simulink model "t2_2_Dinamica_proyectil"  (R2024a)
settings: Solver=VariableStepAuto  StartTime=0.0  StopTime=7  RelTol=1e-3
settings Model: Creator=scpmoxxa  LastModifiedBy=pablo
settings OptimizationCC: ReuseModelBlockBuffer=off
settings DebuggingCC: UnconnectedInputMsg=warning  UnconnectedOutputMsg=warning  UnconnectedLineMsg=warning
settings ModelReferenceCC: EnableRefExpFcnMdlSchedulingChecks=on
settings RTWCC: GPUComputeCapability=3.5  DLArmComputeVersion=19.05

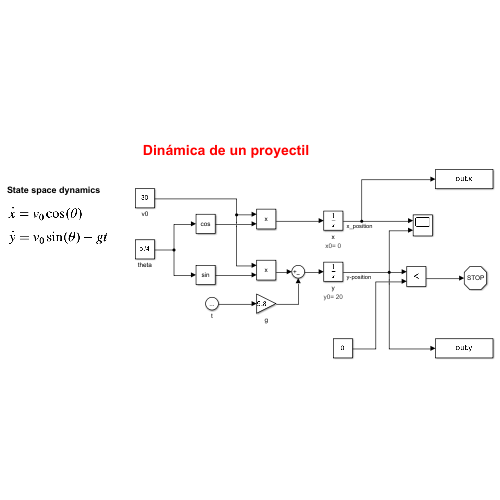
[thumbnail: Simulink's stored preview of the top-level diagram]
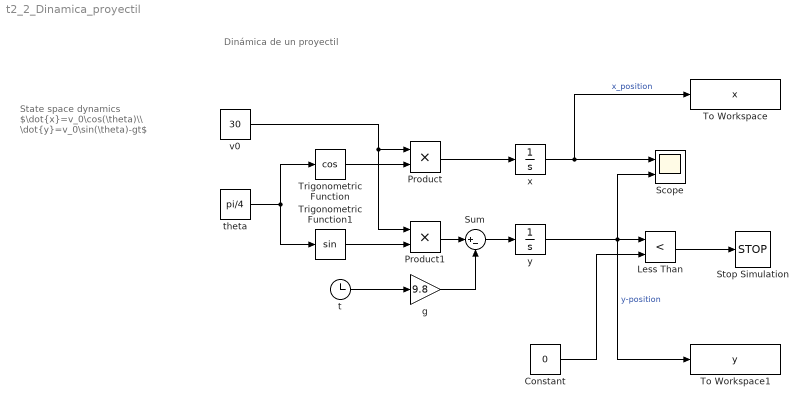
== system t2_2_Dinamica_proyectil ==
  note: State space dynamics
      |
      | $\dot{x}=v_0\cos(\theta)\\ \dot{y}=v_0\sin(\theta)-gt$
  note: Dinámica de un proyectil
  Constant : Constant  Value=0
  Less Than : RelationalOperator  Operator=<  OutDataTypeStr=boolean  RndMeth=Simplest  InputSameDT=off
  Product : Product
  Product1 : Product
  Scope : Scope  NumInputPorts=2
  Stop Simulation : Stop
  Sum : Sum  Inputs=|+-
  To Workspace : ToWorkspace  VariableName=x  SampleTime=-1
  To Workspace1 : ToWorkspace  VariableName=y  SampleTime=-1
  Trigonometric Function : Trigonometry  Operator=cos
  Trigonometric Function1 : Trigonometry
  g : Gain  Gain=9.8
  t : Clock
  theta : Constant  Value=pi/4
  v0 : Constant  Value=30
  x : Integrator
      settings: AttributesFormatString=x0= %<InitialCondition>
  y : Integrator  InitialCondition=20
      settings: AttributesFormatString=y0= %<InitialCondition>
  wires:
  theta/1 -> Trigonometric Function/1, Trigonometric Function1/1
  Trigonometric Function/1 -> Product/2
  v0/1 -> Product1/1, Product/1
  Trigonometric Function1/1 -> Product1/2
  Product/1 -> x/1
  Product1/1 -> Sum/1
  Sum/1 -> y/1
  t/1 -> g/1
  g/1 -> Sum/2
  y/1 -> To Workspace1/1, Scope/2, Less Than/1  "y-position"
  Constant/1 -> Less Than/2
  Less Than/1 -> Stop Simulation/1
  x/1 -> To Workspace/1, Scope/1  "x_position"
